simulink library "brake_lib"  (R2022b)
settings: Solver=VariableStepAuto  StartTime=0.0  StopTime=10.0  RelTol=1e-3
undefined symbols (not defined in the file): raptor_xcp_function
libraries: Raptor_lib x15, simulink x2
settings Model: Creator=serga  LastModifiedBy=serga

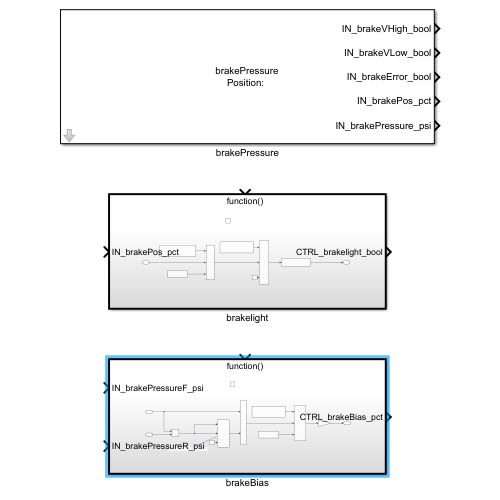
[thumbnail: Simulink's stored preview of the top-level diagram]
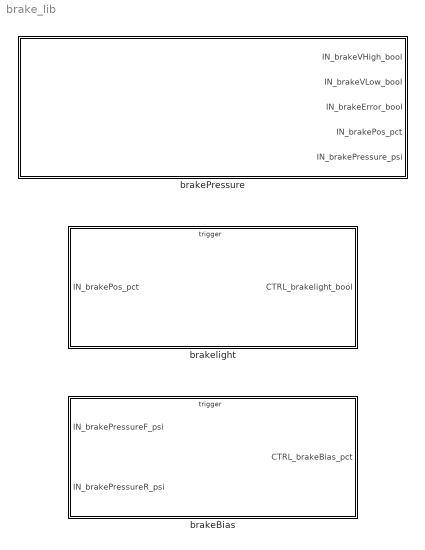
== system brake_lib ==
  brakeBias : Subsystem
  brakePressure : Subsystem  mask{pos=''}
      mask prompts: pos "Position"
      mask Display:
      | disp(['brakePressure\n'...
      |     'Position: ' pos]);
      | port_label('output', 1, ['IN_brakeVHigh' pos '_bool']);
      | port_label('output', 2, ['IN_brakeVLow' pos '_bool']);
      | port_label('output', 3, ['IN_brakeError' pos '_bool']);
      | port_label('output', 4, ['IN_brakePos' pos '_pct']);
      | port_label('output', 5, ['IN_brakePressure' pos '_psi']);
  brakelight : Subsystem

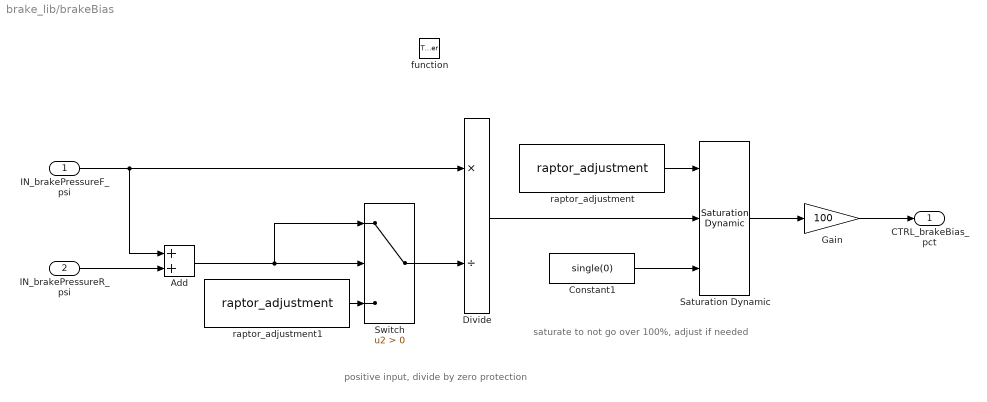
== system brake_lib/brakeBias ==
  note: saturate to not go over 100%, adjust if needed
  note: positive input, divide by zero protection
  IN_brakePressureF_psi : Inport
  IN_brakePressureR_psi : Inport  Port=2
  function : TriggerPort  TriggerType=function-call  VariantControl=(inherit)
  Add : Sum
  Constant1 : Constant  Value=single(0)
  Divide : Product  Inputs=*/
  Gain : Gain  Gain=100
  Saturation Dynamic : simulink/Discontinuities/Saturation Dynamic  OutMin=[]  OutMax=[]  OutDataTypeStr=Inherit: Same as second input  OutDataType=fixdt(1, 16)  OutScaling=2^-10  DoSatur=off
  Switch : Switch  Criteria=u2 > Threshold  SaturateOnIntegerOverflow=off  InputSameDT=off
  raptor_adjustment : Raptor_lib/Data Storage/raptor_adjustment  paramName='CTRL_upperThreshBrakeBias'  nameSource=Parameter  initValue=1  dataType=double  storage=Calibration  calDispType=Number  calEnum={'False', 'True'}  calGain=1.0  calOffset=0.0  calMax=inf  calMin=-inf  calFormat='-1'  calUnit=''  calHelp=''  calAccess=1  calFunction=raptor_xcp_function(gcb)  calDispHeaders=off  calColHeaders={'Col1' 'Col2' 'Col3'}  calRowHeaders={'Row1' 'Row2' 'Row3'}
      settings: SourceProductName=Raptor
  raptor_adjustment1 : Raptor_lib/Data Storage/raptor_adjustment  paramName='CTRL_dbzBrakeBias'  nameSource=Parameter  initValue=1  dataType=single  storage=Calibration  calDispType=Number  calEnum={'False', 'True'}  calGain=1.0  calOffset=0.0  calMax=inf  calMin=-inf  calFormat='-1'  calUnit=''  calHelp=''  calAccess=1  calFunction=raptor_xcp_function(gcb)  calDispHeaders=off  calColHeaders={'Col1' 'Col2' 'Col3'}  calRowHeaders={'Row1' 'Row2' 'Row3'}
      settings: SourceProductName=Raptor
  CTRL_brakeBias_pct : Outport
  wires:
  IN_brakePressureF_psi/1 -> Add/1, Divide/1
  IN_brakePressureR_psi/1 -> Add/2
  Switch/1 -> Divide/2
  raptor_adjustment/1 -> Saturation Dynamic/1
  Constant1/1 -> Saturation Dynamic/3
  Divide/1 -> Saturation Dynamic/2
  Add/1 -> Switch/1, Switch/2
  raptor_adjustment1/1 -> Switch/3
  Saturation Dynamic/1 -> Gain/1
  Gain/1 -> CTRL_brakeBias_pct/1

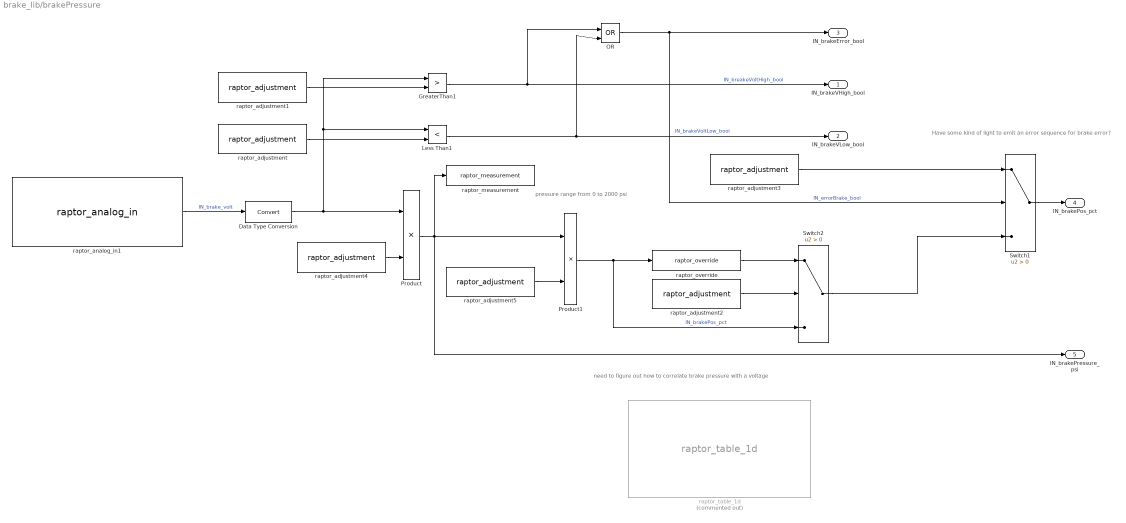
== system brake_lib/brakePressure ==
  note: pressure range from 0 to 2000 psi
  note: need to figure out how to correlate brake pressure with a voltage
  note: Have some kind of light to emit an error sequence for brake error?
  Data Type Conversion : DataTypeConversion  SaturateOnIntegerOverflow=off  RndMeth=Floor
  GreaterThan1 : RelationalOperator  Operator=>  OutDataTypeStr=boolean  RndMeth=Simplest  InputSameDT=off
  Less Than1 : RelationalOperator  Operator=<  OutDataTypeStr=boolean  RndMeth=Simplest  InputSameDT=off
  OR : Logic  Operator=OR  IconShape=distinctive  AllPortsSameDT=off  OutDataTypeStr=boolean
  Product : Product
  Product1 : Product
  Switch1 : Switch  Criteria=u2 > Threshold  SaturateOnIntegerOverflow=off  InputSameDT=off
  Switch2 : Switch  Criteria=u2 > Threshold  SaturateOnIntegerOverflow=off  InputSameDT=off
  raptor_adjustment : Raptor_lib/Data Storage/raptor_adjustment  paramName=['IN_brakeLow' pos '_v']  nameSource=Parameter  initValue=0.5  dataType=single  storage=Calibration  calDispType=Number  calEnum={'False', 'True'}  calGain=1.0  calOffset=0.0  calMax=inf  calMin=-inf  calFormat='-1'  calUnit=''  calHelp=''  calAccess=1  calFunction=raptor_xcp_function(gcb)  calDispHeaders=off  calColHeaders={'Col1' 'Col2' 'Col3'}  calRowHeaders={'Row1' 'Row2' 'Row3'}
      settings: SourceProductName=Raptor
  raptor_adjustment1 : Raptor_lib/Data Storage/raptor_adjustment  paramName=['IN_brakeHigh' pos '_v']  nameSource=Parameter  initValue=4.5  dataType=single  storage=Calibration  calDispType=Number  calEnum={'False', 'True'}  calGain=1.0  calOffset=0.0  calMax=inf  calMin=-inf  calFormat='-1'  calUnit=''  calHelp=''  calAccess=1  calFunction=raptor_xcp_function(gcb)  calDispHeaders=off  calColHeaders={'Col1' 'Col2' 'Col3'}  calRowHeaders={'Row1' 'Row2' 'Row3'}
      settings: SourceProductName=Raptor
  raptor_adjustment2 : Raptor_lib/Data Storage/raptor_adjustment  paramName=['IN_brakePos' pos '_pct']  nameSource=Parameter  initValue=0.00  dataType=boolean  storage=Calibration  calDispType=Number  calEnum={'False', 'True'}  calGain=1.0  calOffset=0.0  calMax=inf  calMin=-inf  calFormat='-1'  calUnit=''  calHelp=''  calAccess=1  calFunction=raptor_xcp_function(gcb)  calDispHeaders=off  calColHeaders={'Col1' 'Col2' 'Col3'}  calRowHeaders={'Row1' 'Row2' 'Row3'}
      settings: SourceProductName=Raptor
  raptor_adjustment3 : Raptor_lib/Data Storage/raptor_adjustment  paramName=['IN_brakePos' pos '_zero']  nameSource=Parameter  initValue=0.00  dataType=boolean  storage=Calibration  calDispType=Number  calEnum={'False', 'True'}  calGain=1.0  calOffset=0.0  calMax=inf  calMin=-inf  calFormat='-1'  calUnit=''  calHelp=''  calAccess=1  calFunction=raptor_xcp_function(gcb)  calDispHeaders=off  calColHeaders={'Col1' 'Col2' 'Col3'}  calRowHeaders={'Row1' 'Row2' 'Row3'}
      settings: SourceProductName=Raptor
  raptor_adjustment4 : Raptor_lib/Data Storage/raptor_adjustment  paramName=['IN_brakePressure' pos '_vToPsi']  nameSource=Parameter  initValue=0.02  dataType=double  storage=Calibration  calDispType=Number  calEnum={'False', 'True'}  calGain=1.0  calOffset=0.0  calMax=inf  calMin=-inf  calFormat='-1'  calUnit=''  calHelp=''  calAccess=1  calFunction=raptor_xcp_function(gcb)  calDispHeaders=off  calColHeaders={'Col1' 'Col2' 'Col3'}  calRowHeaders={'Row1' 'Row2' 'Row3'}
      settings: SourceProductName=Raptor
  raptor_adjustment5 : Raptor_lib/Data Storage/raptor_adjustment  paramName=['IN_brakePressure' pos '_psiToPct']  nameSource=Parameter  initValue=100/2000  dataType=double  storage=Calibration  calDispType=Number  calEnum={'False', 'True'}  calGain=1.0  calOffset=0.0  calMax=inf  calMin=-inf  calFormat='-1'  calUnit=''  calHelp=''  calAccess=1  calFunction=raptor_xcp_function(gcb)  calDispHeaders=off  calColHeaders={'Col1' 'Col2' 'Col3'}  calRowHeaders={'Row1' 'Row2' 'Row3'}
      settings: SourceProductName=Raptor
  raptor_analog_in1 : Raptor_lib/Input & Output/raptor_analog_in  resourceValues=INPUT2|INPUT3|INPUT4|INPUT5|INPUT6|INPUT7|INPUT8|INPUT9|INPUT10|INPUT11|INPUT12|INPUT13|INPUT14|INPUT15|INPUT16|INPUT17|INPUT18|INPUT19|INPUT20|INPUT21|INPUT22|INPUT23|INPUT24|INPUT25|INPUT26|INPUT27|INPUT28|INPUT29|INPUT30|INPUT31|INPUT32|(None)  resource=INPUT3  pullUDValues=2.15k PU  pullUD=2.15k PU  rangeValues=0 - 5 V  range=0 - 5 V  filterrateValues=[]  filterrate='RAPTOR MASK DEFAULT'  resolutionValues=[]  resolution=[]
      settings: SourceProductName=Raptor
  raptor_measurement : Raptor_lib/Data Storage/raptor_measurement  paramName=['IN_brakePressure' pos '_psi']  nameSource=Parameter  calDispType=Number  calEnum={'False', 'True'}  calGain=1.0  calOffset=0.0  calMax=inf  calMin=-inf  calFormat='-1'  calUnit=''  calHelp=''  calAccess=1  calFunction=raptor_xcp_function(gcb)  calVisible=on
      settings: SourceProductName=Raptor
  raptor_override : Raptor_lib/Data Storage/raptor_override  paramName='DataName'  nameSource=Input Wire  measurement=None  calDispType=Number  calEnum={'False', 'True'}  calGain=1.0  calOffset=0.0  calMax=inf  calMin=-inf  calFormat='-1'  calUnit=''  calHelp=''  calAccess=1  calFunction="[raptor_xcp_function(gcb) '|'  'Override']"
      settings: SourceProductName=Raptor
  raptor_table_1d : Raptor_lib/Table Lookup/raptor_table_1d  Commented=on  dataName='IN_brakeToPct'  initValue=[0 10 20 30 40 50 60 70 80 90 100]  dataType=single  storage=Calibration  initValueX=[0.5 0.9 1.3 1.7 2.1 2.5 2.9 3.3 3.7 4.1 4.5]  dataTypeXY=single  storageXY=Calibration  calVisible=on  showTable=on  calGain=1.0  calOffset=0.0  calMax=Inf  calMin=-Inf  calFormat='-1'  calUnit='%'  calHelp=''  showBreakpoint=on  dataNameX=[]  calGainX=1.0  calOffsetX=0.0  calMaxX=Inf  calMinX=-Inf  calFormatX='-1'  calUnitX='V'  calHelpX=''  calAccess=1  calFunction=raptor_xcp_function(gcb)  measureEnable=off  mName=['Data1D_Output']
      settings: SourceProductName=Raptor
  IN_brakeVHigh_bool : Outport  OutDataTypeStr=boolean
  IN_brakeVLow_bool : Outport  Port=2  OutDataTypeStr=boolean
  IN_brakeError_bool : Outport  Port=3  OutDataTypeStr=boolean
  IN_brakePos_pct : Outport  Port=4  OutDataTypeStr=double
  IN_brakePressure_psi : Outport  Port=5  OutDataTypeStr=double
  wires:
  raptor_adjustment1/1 -> GreaterThan1/2
  raptor_adjustment/1 -> Less Than1/2
  raptor_analog_in1/1 -> Data Type Conversion/1  "IN_brake_volt"
  GreaterThan1/1 -> OR/1, IN_brakeVHigh_bool/1  "IN_breakeVoltHigh_bool"
  Less Than1/1 -> OR/2, IN_brakeVLow_bool/1  "IN_brakeVoltLow_bool"
  OR/1 -> Switch1/2, IN_brakeError_bool/1  "IN_errorBrake_bool"
  Switch1/1 -> IN_brakePos_pct/1
  raptor_adjustment3/1 -> Switch1/1
  raptor_adjustment2/1 -> Switch2/2
  raptor_override/1 -> Switch2/1
  Switch2/1 -> Switch1/3
  Product1/1 -> raptor_override/1, Switch2/3  "IN_brakePos_pct"
  Data Type Conversion/1 -> Product/1, GreaterThan1/1, Less Than1/1
  raptor_adjustment4/1 -> Product/2
  Product/1 -> raptor_measurement/1, IN_brakePressure_psi/1, Product1/1
  raptor_adjustment5/1 -> Product1/2

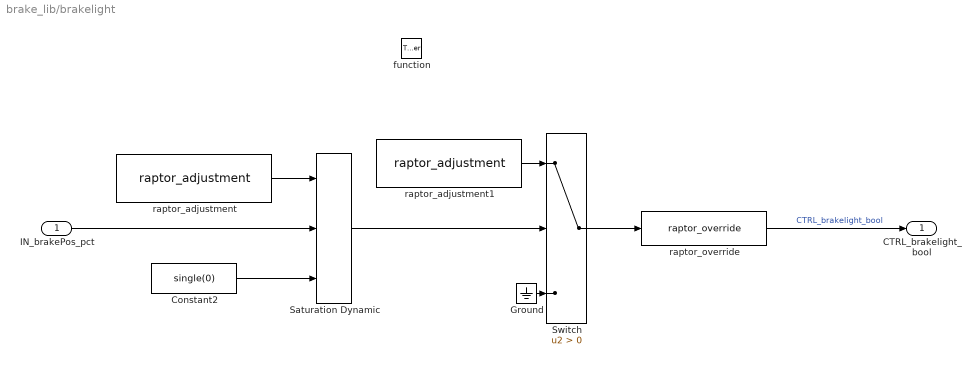
== system brake_lib/brakelight ==
  IN_brakePos_pct : Inport
  function : TriggerPort  TriggerType=function-call  VariantControl=(inherit)
  Constant2 : Constant  Value=single(0)
  Ground : Ground
  Saturation Dynamic : simulink/Discontinuities/Saturation Dynamic  OutMin=[]  OutMax=[]  OutDataTypeStr=Inherit: Same as second input  OutDataType=fixdt(1, 16)  OutScaling=2^-10  DoSatur=off
  Switch : Switch  Criteria=u2 > Threshold  SaturateOnIntegerOverflow=off  InputSameDT=off
  raptor_adjustment : Raptor_lib/Data Storage/raptor_adjustment  paramName='CTRL_upperThreshBrakelight'  nameSource=Parameter  initValue=100  dataType=single  storage=Calibration  calDispType=Number  calEnum={'False', 'True'}  calGain=1.0  calOffset=0.0  calMax=inf  calMin=-inf  calFormat='-1'  calUnit=''  calHelp=''  calAccess=1  calFunction=raptor_xcp_function(gcb)  calDispHeaders=off  calColHeaders={'Col1' 'Col2' 'Col3'}  calRowHeaders={'Row1' 'Row2' 'Row3'}
      settings: SourceProductName=Raptor
  raptor_adjustment1 : Raptor_lib/Data Storage/raptor_adjustment  paramName='CTRL_brakelight_bool'  nameSource=Parameter  initValue=1  dataType=single  storage=Calibration  calDispType=Number  calEnum={'False', 'True'}  calGain=1.0  calOffset=0.0  calMax=inf  calMin=-inf  calFormat='-1'  calUnit=''  calHelp=''  calAccess=1  calFunction=raptor_xcp_function(gcb)  calDispHeaders=off  calColHeaders={'Col1' 'Col2' 'Col3'}  calRowHeaders={'Row1' 'Row2' 'Row3'}
      settings: SourceProductName=Raptor
  raptor_override : Raptor_lib/Data Storage/raptor_override  paramName='DataName'  nameSource=Output Wire  measurement=None  calDispType=Number  calEnum={'False', 'True'}  calGain=1.0  calOffset=0.0  calMax=inf  calMin=-inf  calFormat='-1'  calUnit=''  calHelp=''  calAccess=1  calFunction="[raptor_xcp_function(gcb) '|'  'Override']"
      settings: SourceProductName=Raptor
  CTRL_brakelight_bool : Outport
  wires:
  IN_brakePos_pct/1 -> Saturation Dynamic/2
  raptor_adjustment/1 -> Saturation Dynamic/1
  Constant2/1 -> Saturation Dynamic/3
  Saturation Dynamic/1 -> Switch/2
  raptor_override/1 -> CTRL_brakelight_bool/1  "CTRL_brakelight_bool"
  Switch/1 -> raptor_override/1
  Ground/1 -> Switch/3
  raptor_adjustment1/1 -> Switch/1
